simulink model "projet"  (R2016a)
settings: Solver=VariableStepAuto  StartTime=0.0  StopTime=100.0  RelTol=1e-3
libraries: fuzblock x1
settings Model: Creator=dhiah  LastModifiedBy=dhiah
settings SolverCC: ZeroCrossControl=DisableAll

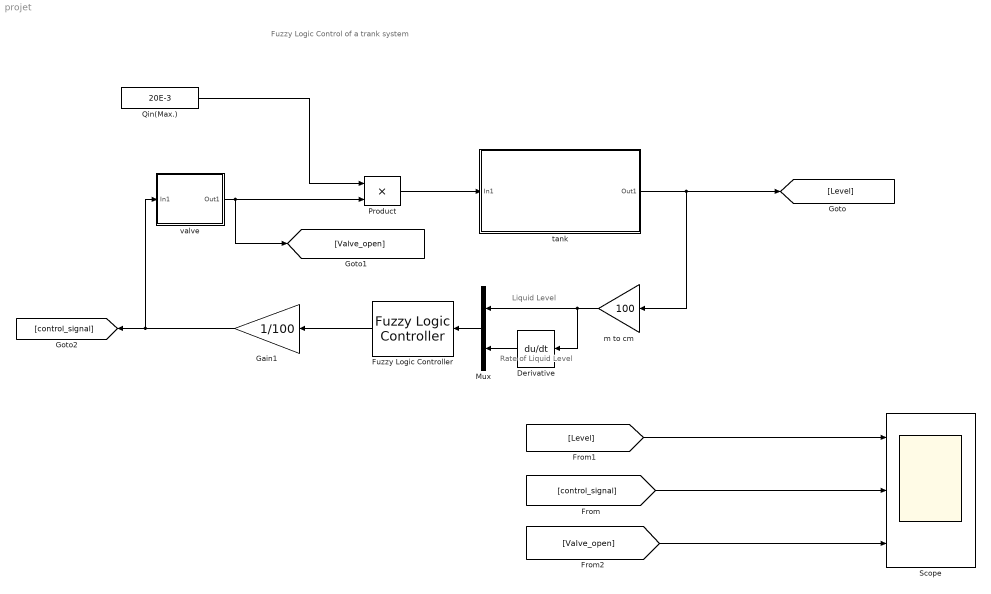
== system projet ==
  note: Fuzzy Logic Control of a trank system
  note: Rate of
      | Liquid Level
  note: Liquid Level
  Derivative : Derivative
  "Fuzzy Logic Controller\t" : fuzblock/Fuzzy Logic  Controller  fis='Trank level system2 5 rules.fis'
  "Gain1 " : Gain  Gain=1/100
  Mux : Mux  Inputs=2
  Product : Product
  Qin(Max.) : Constant  Value=20E-3
  Scope : Scope  NumInputPorts=3
  m to cm : Gain  Gain=100
  tank : Subsystem
      mask Display: image('C:\Users\dhiah\OneDrive\Bureau\projet\trank level system 1.jpg');
  valve : Subsystem
      mask Display: image('C:\Users\dhiah\OneDrive\Bureau\projet\valve.jpg');
  wires:
  Product/1 -> tank/1(In1)
  tank/1(Out1) -> m to cm/1, [Level]
  "Fuzzy Logic Controller\t"/1 -> "Gain1 "/1
  "Gain1 "/1 -> valve/1(In1), [control_signal]
  valve/1(Out1) -> [Valve_open], Product/2
  Qin(Max.)/1 -> Product/1
  Derivative/1 -> Mux/2
  m to cm/1 -> Derivative/1, Mux/1
  Mux/1 -> "Fuzzy Logic Controller\t"/1
  [Level] -> Scope/1
  [control_signal] -> Scope/2
  [Valve_open] -> Scope/3

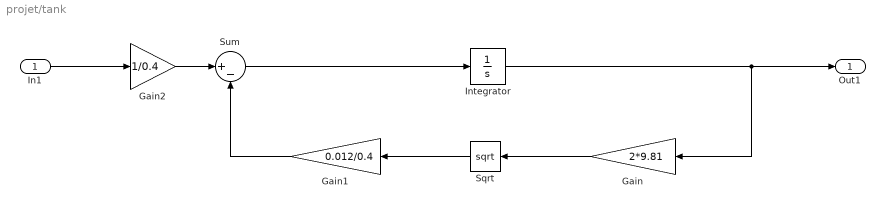
== system projet/tank ==
  In1 : Inport
  Gain : Gain  Gain=2*9.81
  Gain1 : Gain  Gain=0.012/0.4
  Gain2 : Gain  Gain=1/0.4
  Integrator : Integrator
  Sqrt : Sqrt  SaturateOnIntegerOverflow=on
  Sum : Sum  Inputs=|+-
  Out1 : Outport
  wires:
  Sum/1 -> Integrator/1
  Gain2/1 -> Sum/1
  Integrator/1 -> Out1/1, Gain/1
  Gain1/1 -> Sum/2
  Gain/1 -> Sqrt/1
  Sqrt/1 -> Gain1/1
  In1/1 -> Gain2/1

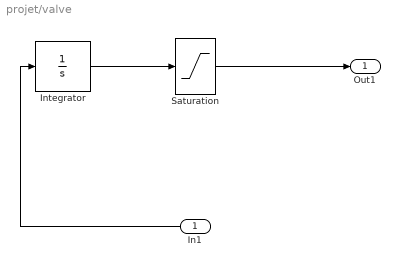
== system projet/valve ==
  In1 : Inport
  Integrator : Integrator
  Saturation : Saturate  UpperLimit=1  LowerLimit=0
  Out1 : Outport
  wires:
  In1/1 -> Integrator/1
  Saturation/1 -> Out1/1
  Integrator/1 -> Saturation/1
